simulink model "InvParkTran"  (R2022b)
settings: Solver=FixedStepDiscrete  StartTime=0.0  StopTime=10.0  FixedStep=0.000001  RelTol=1e-3
settings Model: Creator=yll  LastModifiedBy=yll

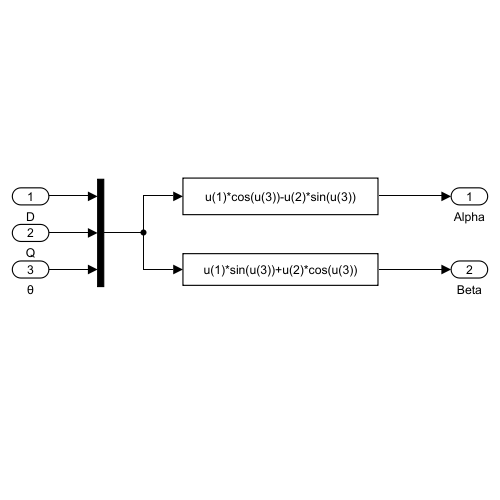
[thumbnail: Simulink's stored preview of the top-level diagram]
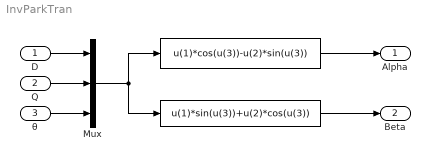
== system InvParkTran ==
  D : Inport
  Q : Inport  Port=2
  θ : Inport  Port=3
  " " : Fcn  Expr=u(1)*cos(u(3))-u(2)*sin(u(3))
  " " : Fcn  Expr=u(1)*sin(u(3))+u(2)*cos(u(3))
  Mux : Mux  Inputs=3
  Alpha : Outport
  Beta : Outport  Port=2
  wires:
  " "/1 -> Beta/1
  D/1 -> Mux/1
  Mux/1 -> " "/1, " "/1
  " "/1 -> Alpha/1
  Q/1 -> Mux/2
  θ/1 -> Mux/3
